simulink model "pacemaker_final"  (R2025a)
settings: Solver=FixedStepAuto  StartTime=0.0  StopTime=10  FixedStep=1e-3  RelTol=1e-3  EnableMultiTasking=on
undefined symbols (not defined in the file): A0, A1, D0, D1, D10, D11, D12, D13, D2, D3, D4, D5, D6, D7, D8, D9, PTA0, PTA1, PTA2, PTB2, PTB23, PTB3, PTB9, PTC16, PTC17, PTC2, PTC3, PTC4, PTD0, PTD1, PTD2, PTD3
libraries: frdmk64flib x20, etargetslib x17, dspstat3 x1
settings Model: ExtModeTrigDuration=5  Creator=School Account  LastModifiedBy=user
settings SolverCC: AlgebraicLoopSolver=TrustRegion
settings OptimizationCC: DefaultParameterBehavior=Inlined  EnhancedBackFolding=on  PassReuseOutputArgsAs=Individual arguments  ZeroExternalMemoryAtStartup=off  ZeroInternalMemoryAtStartup=off  MaxStackSize=64  OptimizeBlockOrder=speed  DifferentSizesBufferReuse=on  OptimizationCustomize=off  EfficientTunableParamExpr=on
settings DebuggingCC: ParameterTunabilityLossMsg=error
settings HardwareCC: ProdBitPerPointer=32.0  ProdBitPerSizeT=32.0  ProdBitPerPtrDiffT=32.0  ProdLargestAtomicInteger=Long  ProdLargestAtomicFloat=Double  ProdWordSize=32.0  ProdHWDeviceType=ARM Compatible->ARM Cortex
settings SFSimCC: MATLABDynamicMemAlloc=off
settings RTWCC: SystemTargetFile=ert.tlc  HardwareBoard=NXP FRDM-K64F  TLCOptions="-aInlineSetEventsForThisBaseRateFcn=TLC_FALSE -aSuppressMultiTaskScheduler=TLC_FALSE  -aRateBasedStepFcn=0"  TemplateMakefile=ert_default_tmf  Toolchain=GNU Tools for ARM Embedded Processors  GPUComputeCapability=3.5  Description=Embedded Coder
settings CodeAppCC: ForceParamTrailComments=on  IgnoreCustomStorageClasses=off  OperatorAnnotations=on  SimulinkDataObjDesc=on  SFDataObjDesc=on  InsertBlockDesc=on
settings ERTTargetCC: ExtModeTransport=4.0  ExtModeStaticAlloc=off  ExtModeMexFile=sendToCommService  ExtModeIntrfLevel=Level1  DynamicArrayContainerType=coder::array

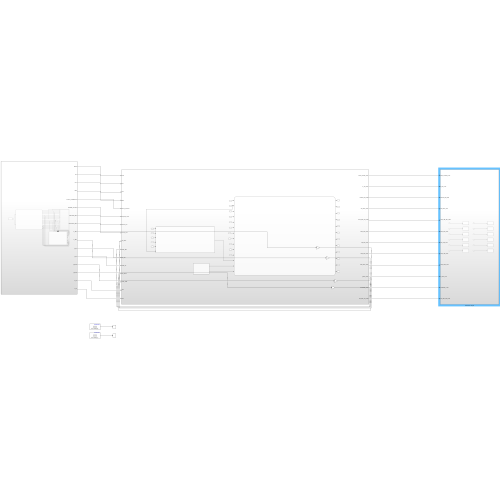
[thumbnail: Simulink's stored preview of the top-level diagram]
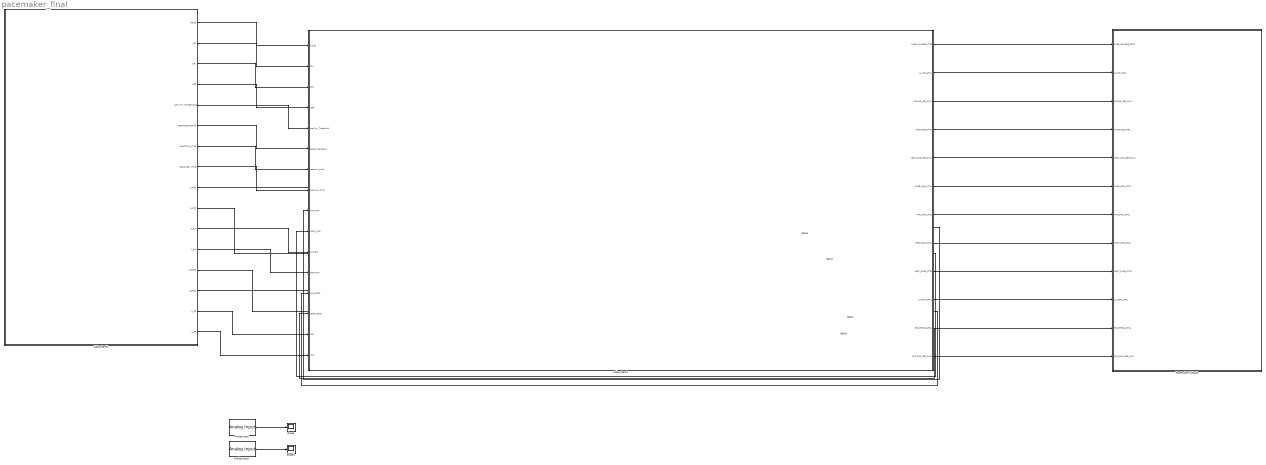
== system pacemaker_final ==
  Analog Input : frdmk64flib/Analog Input  Whichpin=PTB2 (A0)  SampleTime=-1
  Analog Input1 : frdmk64flib/Analog Input  Whichpin=PTB3 (A1)  SampleTime=-1
  Gain1 : Gain  Gain=20
  Gain2 : Gain  Gain=30
  Gain3 : Gain  Gain=30
  Gain4 : Gain  Gain=20
  Pacemaker Outputs : Subsystem
  Scope : Scope
  Scope1 : Scope
      settings: DataLoggingVariableName=ScopeData2
  Subsystem3 : Subsystem
  Subsystem5 : Subsystem
  wires:
  Subsystem3/9(VENT_PACE_CTRL) -> Pacemaker Outputs/9(VENT_PACE_CTRL)
  Subsystem3/8(VENT_GND_CTRL) -> Pacemaker Outputs/8(VENT_GND_CTRL)
  Subsystem3/5(VENT_CMP_REF_PWM) -> Pacemaker Outputs/5(VENT_CMP_REF_PWM)
  Subsystem3/6(PACE_GND_CTRL) -> Pacemaker Outputs/6(PACE_GND_CTRL)
  Subsystem3/3(PACING_REF_PWM) -> Pacemaker Outputs/3(PACING_REF_PWM)
  Subsystem3/4(ATR_PACE_CTRL) -> Pacemaker Outputs/4(ATR_PACE_CTRL)
  Subsystem3/7(ATR_GND_CTRL) -> Pacemaker Outputs/7(ATR_GND_CTRL)
  Subsystem3/10(Z_VENT_CTRL) -> Pacemaker Outputs/10(Z_VENT_CTRL)
  Subsystem3/11(FRONTEND_CTRL) -> Pacemaker Outputs/11(FRONTEND_CTRL)
  Subsystem3/12(ATR_CMP_REF_PWM) -> Pacemaker Outputs/12(ATR_CMP_REF_PWM)
  Subsystem3/1(PACE_CHARGE_CTRL) -> Pacemaker Outputs/1(PACE_CHARGE_CTRL)
  Subsystem3/2(Z_ATR_CTRL) -> Pacemaker Outputs/2(Z_ATR_CTRL)
  Subsystem5/13(A_SENS) -> Gain2/1
  Gain2/1 -> Subsystem3/13(ATR_SENS)
  Subsystem5/9(A_AMP) -> Gain4/1
  Subsystem5/14(V_SENS) -> Gain3/1
  Gain3/1 -> Subsystem3/14(VENT_SENS)
  Subsystem5/11(A_PW) -> Subsystem3/11(ATR_PW)
  Subsystem5/3(URL) -> Subsystem3/3(URL)
  Subsystem5/6(RESPNSE_FACTOR) -> Subsystem3/6(Response_Factor)
  Subsystem5/5(ACTIVITY_THRESHOLD) -> Subsystem3/5(Activity_Threshold)
  Subsystem5/16(V_RP) -> Subsystem3/16(VRP)
  Subsystem5/2(LRL) -> Subsystem3/2(LRL)
  Subsystem5/4(MSR) -> Subsystem3/4(MSR)
  Subsystem5/1(MODE) -> Subsystem3/1(mode)
  Subsystem5/8(RECOVERY_TIME) -> Subsystem3/8(recovery_time)
  Subsystem5/7(REACTION_TIME) -> Subsystem3/7(reaction_time)
  Subsystem5/10(V_AMP) -> Gain1/1
  Gain4/1 -> Subsystem3/9(ATR_AMP)
  Gain1/1 -> Subsystem3/10(VENT_AMP)
  Subsystem5/12(V_PW) -> Subsystem3/12(VENT_PW)
  Subsystem5/15(A_RP) -> Subsystem3/15(ARP)
  Analog Input/1 -> Scope/1
  Analog Input1/1 -> Scope1/1

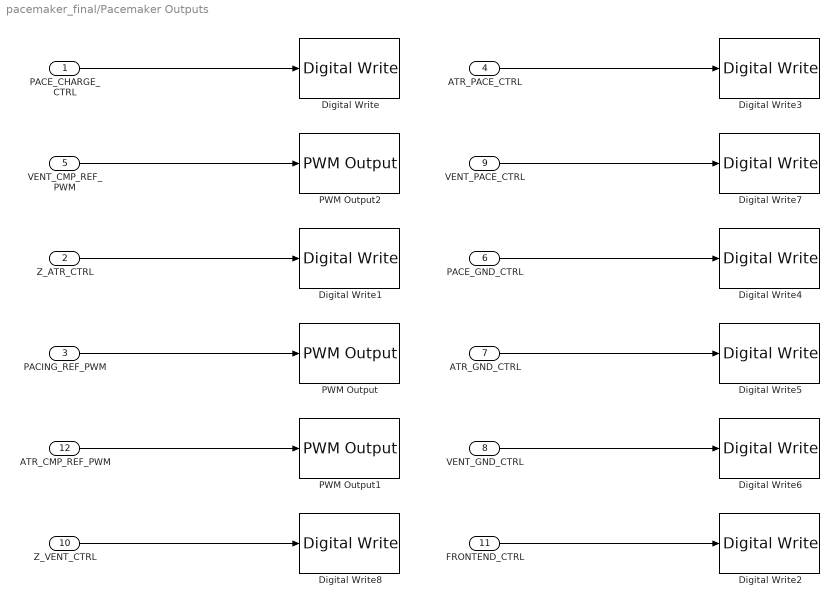
== system pacemaker_final/Pacemaker Outputs ==
  PACE_CHARGE_CTRL : Inport
  Z_ATR_CTRL : Inport  Port=2
  PACING_REF_PWM : Inport  Port=3
  ATR_PACE_CTRL : Inport  Port=4
  VENT_CMP_REF_PWM : Inport  Port=5
  PACE_GND_CTRL : Inport  Port=6
  ATR_GND_CTRL : Inport  Port=7
  VENT_GND_CTRL : Inport  Port=8
  VENT_PACE_CTRL : Inport  Port=9
  Z_VENT_CTRL : Inport  Port=10
  FRONTEND_CTRL : Inport  Port=11
  ATR_CMP_REF_PWM : Inport  Port=12
  Digital Write : frdmk64flib/Digital Write  Whichpin=PTB9 (D2)
  Digital Write1 : frdmk64flib/Digital Write  Whichpin=PTB23 (D4)
  Digital Write2 : frdmk64flib/Digital Write  Whichpin=PTD1 (D13)
  Digital Write3 : frdmk64flib/Digital Write  Whichpin=PTA0 (D8)
  Digital Write4 : frdmk64flib/Digital Write  Whichpin=PTD0 (D10)
  Digital Write5 : frdmk64flib/Digital Write  Whichpin=PTD2 (D11)
  Digital Write6 : frdmk64flib/Digital Write  Whichpin=PTD3 (D12)
  Digital Write7 : frdmk64flib/Digital Write  Whichpin=PTC4 (D9)
  Digital Write8 : frdmk64flib/Digital Write  Whichpin=PTC3 (D7)
  PWM Output : frdmk64flib/PWM Output  Whichpin=PTA2 (D5)  InitialFrequency=2000  InitialDutyCycle=0
  PWM Output1 : frdmk64flib/PWM Output  Whichpin=PTC2 (D6)  InitialFrequency=2000  InitialDutyCycle=0
  PWM Output2 : frdmk64flib/PWM Output  Whichpin=PTA1 (D3)  InitialFrequency=2000  InitialDutyCycle=0
  wires:
  PACE_CHARGE_CTRL/1 -> Digital Write/1
  Z_ATR_CTRL/1 -> Digital Write1/1
  PACING_REF_PWM/1 -> PWM Output/1
  ATR_PACE_CTRL/1 -> Digital Write3/1
  PACE_GND_CTRL/1 -> Digital Write4/1
  ATR_GND_CTRL/1 -> Digital Write5/1
  VENT_GND_CTRL/1 -> Digital Write6/1
  VENT_PACE_CTRL/1 -> Digital Write7/1
  Z_VENT_CTRL/1 -> Digital Write8/1
  FRONTEND_CTRL/1 -> Digital Write2/1
  ATR_CMP_REF_PWM/1 -> PWM Output1/1
  VENT_CMP_REF_PWM/1 -> PWM Output2/1

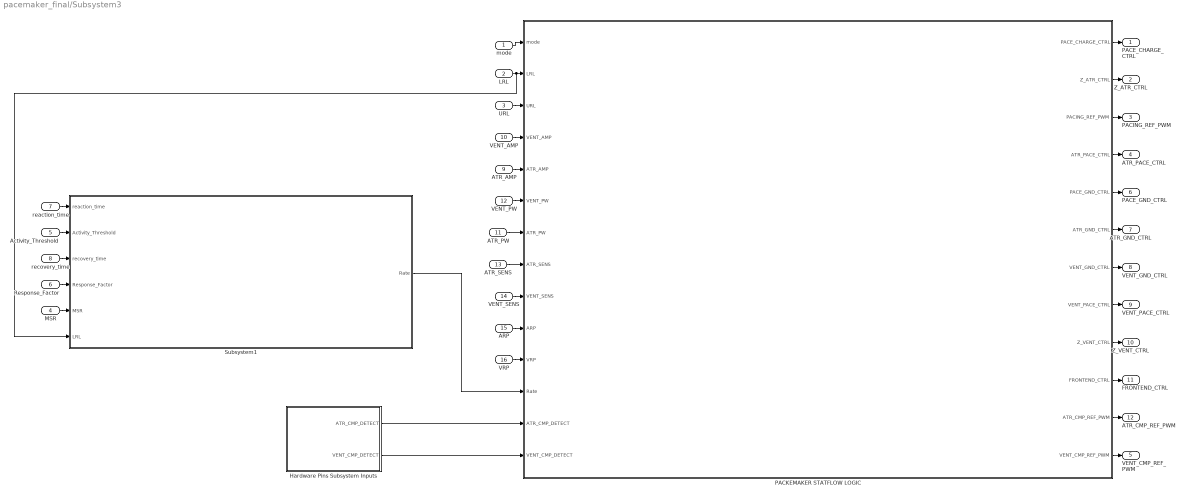
== system pacemaker_final/Subsystem3 ==
  mode : Inport
  LRL : Inport  Port=2
  URL : Inport  Port=3
  MSR : Inport  Port=4
  Activity_Threshold : Inport  Port=5
  Response_Factor : Inport  Port=6
  reaction_time : Inport  Port=7
  recovery_time : Inport  Port=8
  ATR_AMP : Inport  Port=9
  VENT_AMP : Inport  Port=10
  ATR_PW : Inport  Port=11
  VENT_PW : Inport  Port=12
  ATR_SENS : Inport  Port=13
  VENT_SENS : Inport  Port=14
  ARP : Inport  Port=15
  VRP : Inport  Port=16
  Hardware Pins Subsystem Inputs : Subsystem
  PACKEMAKER STATFLOW LOGIC : Stateflow chart  TreatAsAtomicUnit=on
      settings: PortSchema="{\"entries\":[{\"content\":{\"sides\":[{\"content\":{\"connectorIds\":[\"In1\",\"In4\",\"In13\",\"In5\",\"In2\",\"In6\",\"In3\",\"In7\",\"In10\",\"In8\",\"In11\",\"In14\",\"In9\",\"In12\"]},\"type\":\"ConnectorPlacement.EquallySpacedRectSide\",\"uuid\":\"2821f65a-9b3e-4ca7-babd-b0602bfdca31\"},{\"content\":{\"connectorIds\":[\"Out1\",\"Out2\",\"Out3\",\"Out4\",\"Out5\",\"Out6\",\"Out7\",\"Out8\",\"Out9\",\"Out10\",\"Out11\",\"Out12\"],\"side\":\"RIGHT\"},\"type\":\"ConnectorPlacement.EquallySpacedRectSide\",\"uuid\":\"3302ad84-7e85-4bae-9388-240b69681e7f\"},{\"content\":{\"side\":\"TOP\"},\"type\":\"ConnectorPlacement.EquallySpacedRectSide\",\"uuid\":\"cc666da6-1c79-42dc-9f95-9791247ae8bf\"}]},\"type\":\"ConnectorPlacement.EquallySpacedConnector\",\"uuid\":\"e2a43bfa-d126-4f35-adbf-2cf33da0501f\"}],\"packageUris\":[\"http://schema.mathworks.com/mf0/Connector/R2020b\"],\"version\":\"1.0\"}"
  Subsystem1 : Subsystem
  PACE_CHARGE_CTRL : Outport
  Z_ATR_CTRL : Outport  Port=2
  PACING_REF_PWM : Outport  Port=3
  ATR_PACE_CTRL : Outport  Port=4
  VENT_CMP_REF_PWM : Outport  Port=5
  PACE_GND_CTRL : Outport  Port=6
  ATR_GND_CTRL : Outport  Port=7
  VENT_GND_CTRL : Outport  Port=8
  VENT_PACE_CTRL : Outport  Port=9
  Z_VENT_CTRL : Outport  Port=10
  FRONTEND_CTRL : Outport  Port=11
  ATR_CMP_REF_PWM : Outport  Port=12
  wires:
  VENT_PW/1 -> PACKEMAKER STATFLOW LOGIC/6(VENT_PW)
  PACKEMAKER STATFLOW LOGIC/9(Z_VENT_CTRL) -> Z_VENT_CTRL/1
  recovery_time/1 -> Subsystem1/3(recovery_time)
  LRL/1 -> Subsystem1/6(LRL), PACKEMAKER STATFLOW LOGIC/4(LRL)
  PACKEMAKER STATFLOW LOGIC/7(VENT_GND_CTRL) -> VENT_GND_CTRL/1
  Hardware Pins Subsystem Inputs/1(ATR_CMP_DETECT) -> PACKEMAKER STATFLOW LOGIC/9(ATR_CMP_DETECT)
  Response_Factor/1 -> Subsystem1/4(Response_Factor)
  Hardware Pins Subsystem Inputs/2(VENT_CMP_DETECT) -> PACKEMAKER STATFLOW LOGIC/12(VENT_CMP_DETECT)
  Subsystem1/1(Rate) -> PACKEMAKER STATFLOW LOGIC/14(Rate)
  MSR/1 -> Subsystem1/5(MSR)
  PACKEMAKER STATFLOW LOGIC/1(PACE_CHARGE_CTRL) -> PACE_CHARGE_CTRL/1
  Activity_Threshold/1 -> Subsystem1/2(Activity_Threshold)
  PACKEMAKER STATFLOW LOGIC/12(VENT_CMP_REF_PWM) -> VENT_CMP_REF_PWM/1
  PACKEMAKER STATFLOW LOGIC/11(ATR_CMP_REF_PWM) -> ATR_CMP_REF_PWM/1
  reaction_time/1 -> Subsystem1/1(reaction_time)
  PACKEMAKER STATFLOW LOGIC/6(ATR_GND_CTRL) -> ATR_GND_CTRL/1
  PACKEMAKER STATFLOW LOGIC/4(ATR_PACE_CTRL) -> ATR_PACE_CTRL/1
  PACKEMAKER STATFLOW LOGIC/5(PACE_GND_CTRL) -> PACE_GND_CTRL/1
  PACKEMAKER STATFLOW LOGIC/10(FRONTEND_CTRL) -> FRONTEND_CTRL/1
  PACKEMAKER STATFLOW LOGIC/8(VENT_PACE_CTRL) -> VENT_PACE_CTRL/1
  PACKEMAKER STATFLOW LOGIC/3(PACING_REF_PWM) -> PACING_REF_PWM/1
  ATR_SENS/1 -> PACKEMAKER STATFLOW LOGIC/7(ATR_SENS)
  VENT_AMP/1 -> PACKEMAKER STATFLOW LOGIC/5(VENT_AMP)
  ARP/1 -> PACKEMAKER STATFLOW LOGIC/8(ARP)
  VENT_SENS/1 -> PACKEMAKER STATFLOW LOGIC/10(VENT_SENS)
  VRP/1 -> PACKEMAKER STATFLOW LOGIC/11(VRP)
  URL/1 -> PACKEMAKER STATFLOW LOGIC/13(URL)
  PACKEMAKER STATFLOW LOGIC/2(Z_ATR_CTRL) -> Z_ATR_CTRL/1
  mode/1 -> PACKEMAKER STATFLOW LOGIC/1(mode)
  ATR_AMP/1 -> PACKEMAKER STATFLOW LOGIC/2(ATR_AMP)
  ATR_PW/1 -> PACKEMAKER STATFLOW LOGIC/3(ATR_PW)

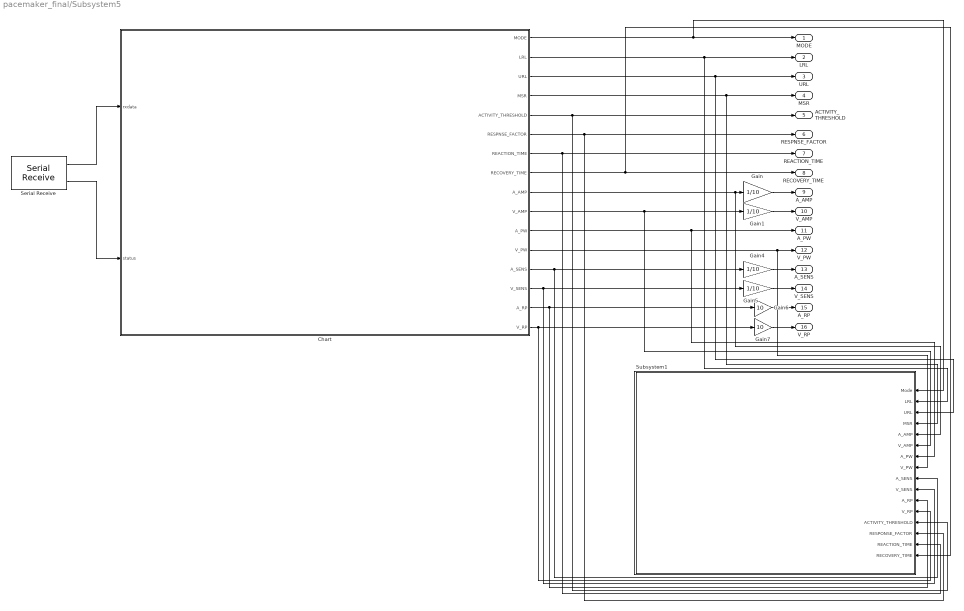
== system pacemaker_final/Subsystem5 ==
  Chart : Stateflow chart  TreatAsAtomicUnit=on
      settings: PortSchema="{\"entries\":[{\"content\":{\"sides\":[{\"content\":{\"connectorIds\":[\"In1\",\"In2\"]},\"type\":\"ConnectorPlacement.EquallySpacedRectSide\",\"uuid\":\"7451ee94-9b00-43e8-b3be-cdc332c766dc\"},{\"content\":{\"connectorIds\":[\"Out6\",\"Out5\",\"Out12\",\"Out7\",\"Out9\",\"Out11\",\"Out8\",\"Out10\",\"Out1\",\"Out13\",\"Out2\",\"Out14\",\"Out4\",\"Out16\",\"Out3\",\"Out15\"],\"side\":\"RIGHT\"},\"type\":\"ConnectorPlacement.EquallySpacedRectSide\",\"uuid\":\"f2d3f72a-cf0a-47d0-b806-afde7d262d5f\"},{\"content\":{\"side\":\"TOP\"},\"type\":\"ConnectorPlacement.EquallySpacedRectSide\",\"uuid\":\"0a90c947-4341-46b5-8896-9140e37675a1\"}]},\"type\":\"ConnectorPlacement.EquallySpacedConnector\",\"uuid\":\"30257972-17b0-4b0b-bedd-1116085aa9d3\"}],\"packageUris\":[\"http://schema.mathworks.com/mf0/Connector/R2020b\"],\"version\":\"1.0\"}"
  Gain{,1,4..5} (4 alike) : Gain  Gain=1/10
  Gain6 : Gain  Gain=10
  Gain7 : Gain  Gain=10
  Serial Receive : frdmk64flib/Serial Receive  SCIModule=0  Baudrate=uint32(9600)  Parity=None  StopBits=1  HardwareFlowControl=None  ByteOrder=LittleEndian  DataType=uint8  DataLength=18  BlockingMode=off  OutputStatus=on  SampleTime=-1
  Subsystem1 : Subsystem
  MODE : Outport
  LRL : Outport  Port=2
  URL : Outport  Port=3
  MSR : Outport  Port=4
  ACTIVITY_THRESHOLD : Outport  Port=5
  RESPNSE_FACTOR : Outport  Port=6
  REACTION_TIME : Outport  Port=7
  RECOVERY_TIME : Outport  Port=8
  A_AMP : Outport  Port=9
  V_AMP : Outport  Port=10
  A_PW : Outport  Port=11
  V_PW : Outport  Port=12
  A_SENS : Outport  Port=13
  V_SENS : Outport  Port=14
  A_RP : Outport  Port=15
  V_RP : Outport  Port=16
  wires:
  Chart/16(V_SENS) -> Subsystem1/10(V_SENS), Gain5/1
  Chart/13(V_AMP) -> Subsystem1/6(V_AMP), Gain1/1
  Chart/1(A_AMP) -> Subsystem1/5(A_AMP), Gain/1
  Serial Receive/1 -> Chart/1(rxdata)
  Chart/3(A_RP) -> Subsystem1/11(A_RP), Gain6/1
  Gain7/1 -> V_RP/1
  Chart/4(A_SENS) -> Subsystem1/9(A_SENS), Gain4/1
  Gain5/1 -> V_SENS/1
  Chart/10(RECOVERY_TIME) -> Subsystem1/16(RECOVERY_TIME), RECOVERY_TIME/1
  Chart/15(V_RP) -> Subsystem1/12(V_RP), Gain7/1
  Chart/2(A_PW) -> A_PW/1, Subsystem1/7(A_PW)
  Chart/11(RESPNSE_FACTOR) -> Subsystem1/14(RESPONSE_FACTOR), RESPNSE_FACTOR/1
  Chart/6(MODE) -> Subsystem1/1(Mode), MODE/1
  Chart/5(LRL) -> Subsystem1/2(LRL), LRL/1
  Chart/9(ACTIVITY_THRESHOLD) -> Subsystem1/13(ACTIVITY_THRESHOLD), ACTIVITY_THRESHOLD/1
  Gain1/1 -> V_AMP/1
  Gain6/1 -> A_RP/1
  Chart/7(MSR) -> Subsystem1/4(MSR), MSR/1
  Chart/14(V_PW) -> V_PW/1, Subsystem1/8(V_PW)
  Chart/12(URL) -> Subsystem1/3(URL), URL/1
  Gain4/1 -> A_SENS/1
  Gain/1 -> A_AMP/1
  Chart/8(REACTION_TIME) -> Subsystem1/15(REACTION_TIME), REACTION_TIME/1
  Serial Receive/2 -> Chart/2(status)

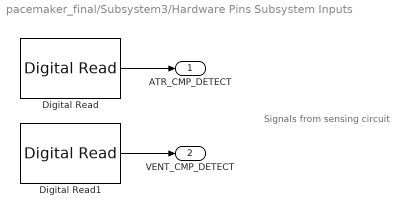
== system pacemaker_final/Subsystem3/Hardware Pins Subsystem Inputs ==
  note: Signals from sensing circuit
  Digital Read : frdmk64flib/Digital Read  Whichpin=PTC16 (D0)  SampleTime=-1
  Digital Read1 : frdmk64flib/Digital Read  Whichpin=PTC17 (D1)  SampleTime=-1
  ATR_CMP_DETECT : Outport
  VENT_CMP_DETECT : Outport  Port=2
  wires:
  Digital Read1/1 -> VENT_CMP_DETECT/1
  Digital Read/1 -> ATR_CMP_DETECT/1

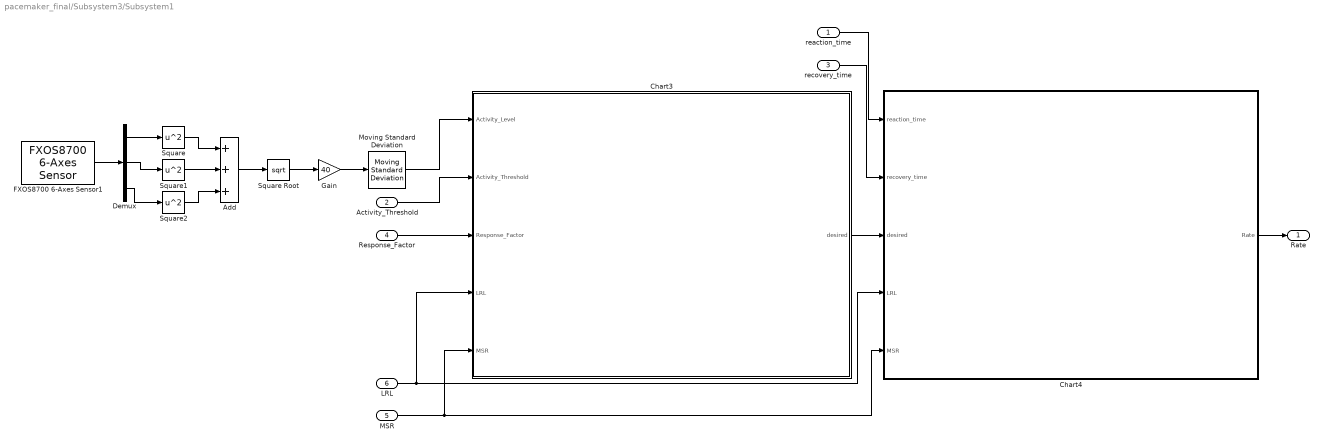
== system pacemaker_final/Subsystem3/Subsystem1 ==
  reaction_time : Inport
  Activity_Threshold : Inport  Port=2
  recovery_time : Inport  Port=3
  Response_Factor : Inport  Port=4
  MSR : Inport  Port=5
  LRL : Inport  Port=6
  Add : Sum  Inputs=+++
  Chart3 : Stateflow chart  TreatAsAtomicUnit=on
  Chart4 : Stateflow chart  TreatAsAtomicUnit=on
      settings: PortSchema="{\"entries\":[{\"content\":{\"sides\":[{\"content\":{\"connectorIds\":[\"In2\",\"In3\",\"In1\",\"In4\",\"In5\"]},\"type\":\"ConnectorPlacement.EquallySpacedRectSide\",\"uuid\":\"edd6887c-315a-49b4-96c6-4b9a398dbb27\"},{\"content\":{\"connectorIds\":[\"Out1\"],\"side\":\"RIGHT\"},\"type\":\"ConnectorPlacement.EquallySpacedRectSide\",\"uuid\":\"e866e153-969a-414b-b9d6-9523e8ffb3f5\"},{\"content\":{\"side\":\"TOP\"},\"type\":\"ConnectorPlacement.EquallySpacedRectSide\",\"uuid\":\"a76f5b9a-cc35-4ca0-a576-c8c761db09b7\"}]},\"type\":\"ConnectorPlacement.EquallySpacedConnector\",\"uuid\":\"7226b5a5-c660-4be3-8454-fc3b1c597f0f\"}],\"packageUris\":[\"http://schema.mathworks.com/mf0/Connector/R2020b\"],\"version\":\"1.0\"}"
  Demux : Demux  Outputs=3
  FXOS8700 6-Axes Sensor1 : frdmk64flib/FXOS8700 6-Axes Sensor  Activesensor=Accelerometer only  ODR=800Hz  HybridODR=400Hz  Accelfullrange=-4g to +4g  SampleTime=0.01
  Gain : Gain  Gain=40
  Moving Standard Deviation : dspstat3/Moving Standard Deviation  Method=Sliding window  ForgettingFactorPort=off  SpecifyWindowLength=on  WindowLength=128  OverlapLength=127  AllowArbitraryInputLength=off  ForgettingFactor=0.9  SimulateUsing=Interpreted execution
  Square : Math  Operator=square
  Square Root : Sqrt
  Square1 : Math  Operator=square
  Square2 : Math  Operator=square
  Rate : Outport
  wires:
  FXOS8700 6-Axes Sensor1/1 -> Demux/1
  Add/1 -> Square Root/1
  Demux/1 -> Square/1
  Demux/2 -> Square1/1
  MSR/1 -> Chart4/5(MSR), Chart3/5(MSR)
  Demux/3 -> Square2/1
  Chart3/1(desired) -> Chart4/1(desired)
  Square/1 -> Add/1
  Square1/1 -> Add/2
  Square2/1 -> Add/3
  Square Root/1 -> Gain/1
  Gain/1 -> Moving Standard Deviation/1
  recovery_time/1 -> Chart4/3(recovery_time)
  Moving Standard Deviation/1 -> Chart3/1(Activity_Level)
  reaction_time/1 -> Chart4/2(reaction_time)
  Activity_Threshold/1 -> Chart3/2(Activity_Threshold)
  Response_Factor/1 -> Chart3/3(Response_Factor)
  LRL/1 -> Chart4/4(LRL), Chart3/4(LRL)
  Chart4/1(Rate) -> Rate/1

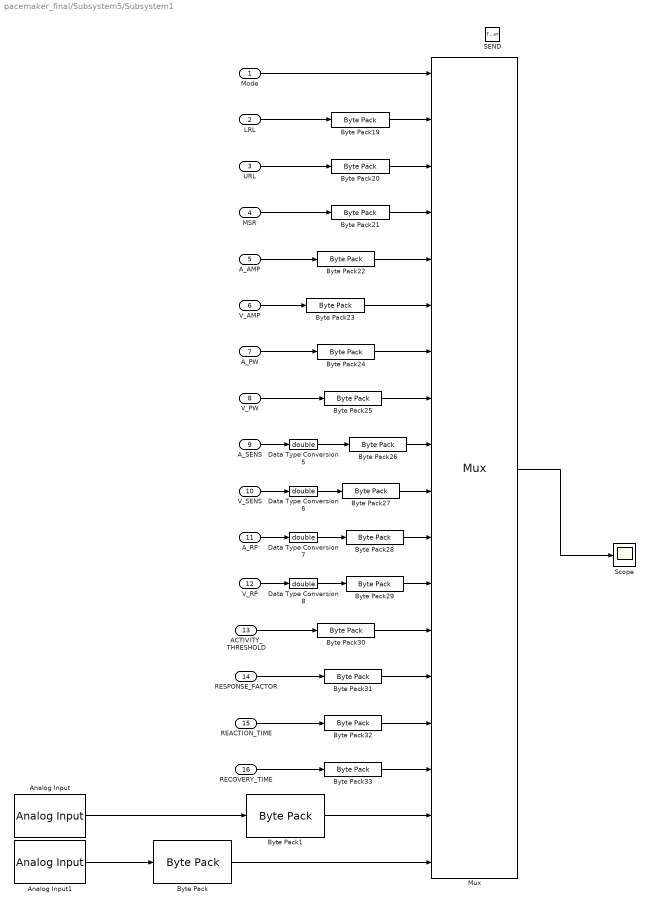
== system pacemaker_final/Subsystem5/Subsystem1 ==
  Mode : Inport
  LRL : Inport  Port=2
  URL : Inport  Port=3
  MSR : Inport  Port=4
  A_AMP : Inport  Port=5
  V_AMP : Inport  Port=6
  A_PW : Inport  Port=7
  V_PW : Inport  Port=8
  A_SENS : Inport  Port=9
  V_SENS : Inport  Port=10
  A_RP : Inport  Port=11
  V_RP : Inport  Port=12
  ACTIVITY_THRESHOLD : Inport  Port=13
  RESPONSE_FACTOR : Inport  Port=14
  REACTION_TIME : Inport  Port=15
  RECOVERY_TIME : Inport  Port=16
  SEND : TriggerPort  TriggerType=function-call  IsSimulinkFunction=on  FunctionName=SEND_PARAM  VariantControl=(inherit)
  Analog Input : frdmk64flib/Analog Input  Whichpin=PTB3 (A1)  SampleTime=-1
  Analog Input1 : frdmk64flib/Analog Input  Whichpin=PTB2 (A0)  SampleTime=-1
  Byte Pack{,1,19..33} (17 alike) : etargetslib/Byte Pack  datatypes={'double'}  byteAlign=1
  Data Type Conversion{5..8} (4 alike) : DataTypeConversion  OutDataTypeStr=double  SaturateOnIntegerOverflow=off  RndMeth=Floor
  Mux : Mux  Inputs=18
  Scope : Scope
  wires:
  Mode/1 -> Mux/1
  Mux/1 -> Scope/1
  LRL/1 -> Byte Pack19/1
  URL/1 -> Byte Pack20/1
  A_AMP/1 -> Byte Pack22/1
  V_AMP/1 -> Byte Pack23/1
  MSR/1 -> Byte Pack21/1
  A_RP/1 -> Data Type Conversion7/1
  V_PW/1 -> Byte Pack25/1
  V_SENS/1 -> Data Type Conversion6/1
  A_SENS/1 -> Data Type Conversion5/1
  A_PW/1 -> Byte Pack24/1
  V_RP/1 -> Data Type Conversion8/1
  RESPONSE_FACTOR/1 -> Byte Pack31/1
  RECOVERY_TIME/1 -> Byte Pack33/1
  REACTION_TIME/1 -> Byte Pack32/1
  ACTIVITY_THRESHOLD/1 -> Byte Pack30/1
  Byte Pack1/1 -> Mux/17
  Analog Input1/1 -> Byte Pack/1
  Byte Pack/1 -> Mux/18
  Analog Input/1 -> Byte Pack1/1
  Byte Pack19/1 -> Mux/2
  Byte Pack20/1 -> Mux/3
  Byte Pack21/1 -> Mux/4
  Byte Pack22/1 -> Mux/5
  Byte Pack23/1 -> Mux/6
  Byte Pack24/1 -> Mux/7
  Byte Pack25/1 -> Mux/8
  Byte Pack26/1 -> Mux/9
  Data Type Conversion5/1 -> Byte Pack26/1
  Data Type Conversion6/1 -> Byte Pack27/1
  Data Type Conversion7/1 -> Byte Pack28/1
  Data Type Conversion8/1 -> Byte Pack29/1
  Byte Pack27/1 -> Mux/10
  Byte Pack28/1 -> Mux/11
  Byte Pack29/1 -> Mux/12
  Byte Pack30/1 -> Mux/13
  Byte Pack31/1 -> Mux/14
  Byte Pack32/1 -> Mux/15
  Byte Pack33/1 -> Mux/16

== stateflow chart pacemaker_final/Subsystem3/PACKEMAKER STATFLOW LOGIC ==
  state Start
  state AOO
    state AOO_Charge
      entry:
      %Charging C22
      ATR_PACE_CTRL = 0;
      VENT_PACE_CTRL = 0;
      PACING_REF_PWM = ATR_AMP;
      PACE_CHARGE_CTRL = 1;
      %Discharging C21
      PACE_GND_CTRL = 1;
      ATR_PACE_CTRL = 0;
      Z_VENT_CTRL = 0;
      Z_ATR_CTRL = 0;
      VENT_PACE_CTRL = 0;
      VENT_GND_CTRL = 0;
      ATR_GND_CTRL = 1;
    state AOO_Pace
      entry:
      %Pacing
      PACE_CHARGE_CTRL = 0;
      PACE_GND_CTRL= 1;
      VENT_PACE_CTRL = 0;
      VENT_GND_CTRL= 0;
      Z_VENT_CTRL = 0;
      Z_ATR_CTRL = 0;
      ATR_GND_CTRL = 0;
      ATR_PACE_CTRL = 1;
    (default) -> AOO.AOO_Charge
    AOO.AOO_Charge -> AOO.AOO_Pace : [after(60000/LRL - ATR_PW,msec)]
    AOO.AOO_Pace -> AOO.AOO_Charge : [after(ATR_PW,msec)]
  state VOO
    state VOO_Charge
      entry:
      %Charging C22
      VENT_PACE_CTRL = 0;
      ATR_PACE_CTRL = 0;
      PACING_REF_PWM = VENT_AMP;
      PACE_CHARGE_CTRL = 1;
      %Discharging C21
      PACE_GND_CTRL = 1;
      VENT_PACE_CTRL = 0;
      Z_ATR_CTRL = 0;
      Z_VENT_CTRL = 0;
      ATR_PACE_CTRL = 0;
      ATR_GND_CTRL = 0;
      VENT_GND_CTRL = 1;
    state AOO_Pace
      entry:
      %Pacing
      PACE_CHARGE_CTRL = 0;
      PACE_GND_CTRL= 1;
      ATR_PACE_CTRL = 0;
      ATR_GND_CTRL= 0;
      Z_ATR_CTRL = 0;
      Z_VENT_CTRL = 0;
      VENT_GND_CTRL = 0;
      VENT_PACE_CTRL = 1;
    (default) -> VOO.VOO_Charge
    VOO.VOO_Charge -> VOO.AOO_Pace : [after(60000/LRL  - VENT_PW,msec)]
    VOO.AOO_Pace -> VOO.VOO_Charge : [after(VENT_PW,msec)]
  state AAI
    state AAI_Charge
      entry:
      FRONTEND_CTRL = 1;
      %Charging C22
      ATR_PACE_CTRL = 0;
      VENT_PACE_CTRL = 0;
      PACING_REF_PWM = ATR_AMP;
      PACE_CHARGE_CTRL = 1;
      %Discharging C21
      PACE_GND_CTRL = 1;
      ATR_PACE_CTRL = 0;
      Z_VENT_CTRL = 0;
      Z_ATR_CTRL = 0;
      VENT_PACE_CTRL = 0;
      VENT_GND_CTRL = 0;
      ATR_GND_CTRL = 1;
      ATR_CMP_REF_PWM = ATR_SENS;
    state AAI_Pace
      entry:
      FRONTEND_CTRL = 0;
      %Pacing
      PACE_CHARGE_CTRL = 0;
      PACE_GND_CTRL= 1;
      VENT_PACE_CTRL = 0;
      VENT_GND_CTRL= 0;
      Z_VENT_CTRL = 0;
      Z_ATR_CTRL = 0;
      ATR_GND_CTRL = 0;
      ATR_PACE_CTRL= 1;
    (default) -> AAI.AAI_Charge
    AAI.AAI_Charge -> AAI.AAI_Pace [order 1] : [after(60000/LRL  - ATR_PW - ARP,msec)]
    AAI.AAI_Pace -> AAI.AAI_Charge : [after( ATR_PW,msec)]
    AAI.AAI_Charge -> (junction 58) [order 2] : [ATR_CMP_DETECT == 1]
    (junction 58) -> (junction 84) : [after(ATR_PW,msec)]
    (junction 84) -> AAI.AAI_Charge : [after(ARP, msec)]
  state VVI
    state VVI_Charge
      entry:
      FRONTEND_CTRL = 1;
      %Charging C22
      VENT_PACE_CTRL = 0;
      ATR_PACE_CTRL = 0;
      PACING_REF_PWM = VENT_AMP;
      PACE_CHARGE_CTRL = 1;
      %Discharging C21
      PACE_GND_CTRL = 1;
      VENT_PACE_CTRL = 0;
      Z_ATR_CTRL = 0;
      Z_VENT_CTRL = 0;
      ATR_PACE_CTRL = 0;
      ATR_GND_CTRL = 0;
      VENT_GND_CTRL = 1;
      VENT_CMP_REF_PWM = VENT_SENS;
    state VVI_Pace
      entry:
      FRONTEND_CTRL = 0;
      %Pacing
      PACE_CHARGE_CTRL = 0;
      PACE_GND_CTRL= 1;
      ATR_PACE_CTRL = 0;
      ATR_GND_CTRL= 0;
      Z_ATR_CTRL = 0;
      Z_VENT_CTRL = 0;
      VENT_GND_CTRL = 0;
      VENT_PACE_CTRL = 1;
    (default) -> VVI.VVI_Charge
    VVI.VVI_Charge -> VVI.VVI_Pace [order 1] : [after(60000/LRL  - VENT_PW - VRP,msec)]
    VVI.VVI_Pace -> VVI.VVI_Charge : [after(VENT_PW,msec)]
    VVI.VVI_Charge -> (junction 65) [order 2] : [VENT_CMP_DETECT == 1]
    (junction 65) -> (junction 82) : [after(VENT_PW,msec)]
    (junction 82) -> VVI.VVI_Charge : [after(VRP, msec)]
  state AOOR
    state AOO_Charge
      entry:
      %Charging C22
      ATR_PACE_CTRL = 0;
      VENT_PACE_CTRL = 0;
      PACING_REF_PWM = ATR_AMP;
      PACE_CHARGE_CTRL = 1;
      %Discharging C21
      PACE_GND_CTRL = 1;
      ATR_PACE_CTRL = 0;
      Z_VENT_CTRL = 0;
      Z_ATR_CTRL = 0;
      VENT_PACE_CTRL = 0;
      VENT_GND_CTRL = 0;
      ATR_GND_CTRL = 1;
    state AOO_Pace
      entry:
      %Pacing
      PACE_CHARGE_CTRL = 0;
      PACE_GND_CTRL= 1;
      VENT_PACE_CTRL = 0;
      VENT_GND_CTRL= 0;
      Z_VENT_CTRL = 0;
      Z_ATR_CTRL = 0;
      ATR_GND_CTRL = 0;
      ATR_PACE_CTRL = 1;
    (default) -> AOOR.AOO_Charge
    AOOR.AOO_Charge -> AOOR.AOO_Pace : [after(60000/Rate - ATR_PW,msec)]
    AOOR.AOO_Pace -> AOOR.AOO_Charge : [after(ATR_PW,msec)]
  state VOOR
    state VOO_Charge
      entry:
      %Charging C22
      VENT_PACE_CTRL = 0;
      ATR_PACE_CTRL = 0;
      PACING_REF_PWM = VENT_AMP;
      PACE_CHARGE_CTRL = 1;
      %Discharging C21
      PACE_GND_CTRL = 1;
      VENT_PACE_CTRL = 0;
      Z_ATR_CTRL = 0;
      Z_VENT_CTRL = 0;
      ATR_PACE_CTRL = 0;
      ATR_GND_CTRL = 0;
      VENT_GND_CTRL = 1;
    state AOO_Pace
      entry:
      %Pacing
      PACE_CHARGE_CTRL = 0;
      PACE_GND_CTRL= 1;
      ATR_PACE_CTRL = 0;
      ATR_GND_CTRL= 0;
      Z_ATR_CTRL = 0;
      Z_VENT_CTRL = 0;
      VENT_GND_CTRL = 0;
      VENT_PACE_CTRL = 1;
    (default) -> VOOR.VOO_Charge
    VOOR.VOO_Charge -> VOOR.AOO_Pace : [after(60000/Rate - VENT_PW,msec)]
    VOOR.AOO_Pace -> VOOR.VOO_Charge : [after(VENT_PW,msec)]
  state AAIR
    state AAI_Charge
      entry:
      FRONTEND_CTRL = 1;
      %Charging C22
      ATR_PACE_CTRL = 0;
      VENT_PACE_CTRL = 0;
      PACING_REF_PWM = ATR_AMP;
      PACE_CHARGE_CTRL = 1;
      %Discharging C21
      PACE_GND_CTRL = 1;
      ATR_PACE_CTRL = 0;
      Z_VENT_CTRL = 0;
      Z_ATR_CTRL = 0;
      VENT_PACE_CTRL = 0;
      VENT_GND_CTRL = 0;
      ATR_GND_CTRL = 1;
      ATR_CMP_REF_PWM = ATR_SENS;
    state AAI_Pace
      entry:
      FRONTEND_CTRL = 0;
      %Pacing
      PACE_CHARGE_CTRL = 0;
      PACE_GND_CTRL= 1;
      VENT_PACE_CTRL = 0;
      VENT_GND_CTRL= 0;
      Z_VENT_CTRL = 0;
      Z_ATR_CTRL = 0;
      ATR_GND_CTRL = 0;
      ATR_PACE_CTRL= 1;
    (default) -> AAIR.AAI_Charge
    AAIR.AAI_Charge -> AAIR.AAI_Pace [order 1] : [after(60000/Rate - ATR_PW - ARP,msec)]
    AAIR.AAI_Pace -> AAIR.AAI_Charge : [after( ATR_PW,msec)]
    AAIR.AAI_Charge -> (junction 107) [order 2] : [ATR_CMP_DETECT == 1]
    (junction 107) -> (junction 108) : [after(ATR_PW,msec)]
    (junction 108) -> AAIR.AAI_Charge : [after(ARP, msec)]
  state VVIR
    state VVI_Charge
      entry:
      FRONTEND_CTRL = 1;
      %Charging C22
      VENT_PACE_CTRL = 0;
      ATR_PACE_CTRL = 0;
      PACING_REF_PWM = VENT_AMP;
      PACE_CHARGE_CTRL = 1;
      %Discharging C21
      PACE_GND_CTRL = 1;
      VENT_PACE_CTRL = 0;
      Z_ATR_CTRL = 0;
      Z_VENT_CTRL = 0;
      ATR_PACE_CTRL = 0;
      ATR_GND_CTRL = 0;
      VENT_GND_CTRL = 1;
      VENT_CMP_REF_PWM = VENT_SENS;
    state VVI_Pace
      entry:
      FRONTEND_CTRL = 0;
      %Pacing
      PACE_CHARGE_CTRL = 0;
      PACE_GND_CTRL= 1;
      ATR_PACE_CTRL = 0;
      ATR_GND_CTRL= 0;
      Z_ATR_CTRL = 0;
      Z_VENT_CTRL = 0;
      VENT_GND_CTRL = 0;
      VENT_PACE_CTRL = 1;
    (default) -> VVIR.VVI_Charge
    VVIR.VVI_Charge -> VVIR.VVI_Pace [order 1] : [after(60000/Rate - VENT_PW - VRP,msec)]
    VVIR.VVI_Pace -> VVIR.VVI_Charge : [after(VENT_PW,msec)]
    VVIR.VVI_Charge -> (junction 118) [order 2] : [VENT_CMP_DETECT == 1]
    (junction 118) -> (junction 119) : [after(VENT_PW,msec)]
    (junction 119) -> VVIR.VVI_Charge : [after(VRP, msec)]
  (default) -> Start
  AOO -> Start : [mode ~= 1]
  Start -> AOO [order 2] : [mode == 1]
  Start -> VOO [order 1] : [mode == 2]
  VOO -> Start : [mode ~= 2]
  Start -> AAI [order 3] : [mode == 3]
  AAI -> Start : [mode ~= 3]
  Start -> VVI [order 4] : [mode == 4]
  VVI -> Start : [mode ~= 4]
  Start -> AOOR [order 5] : [mode == 5]
  AOOR -> Start : [mode ~= 5]
  Start -> VOOR [order 6] : [mode == 6]
  VOOR -> Start : [mode ~= 6]
  Start -> AAIR [order 7] : [mode == 7]
  AAIR -> Start : [mode ~= 7]
  Start -> VVIR [order 8] : [mode == 8]
  VVIR -> Start : [mode ~= 8]
  data: PACE_CHARGE_CTRL output; Z_ATR_CTRL output; PACING_REF_PWM output; mode input; ATR_PACE_CTRL output; PACE_GND_CTRL output; ATR_AMP input; ATR_GND_CTRL output; ATR_PW input; LRL input; VENT_AMP input; VENT_GND_CTRL output; VENT_PACE_CTRL output; Z_VENT_CTRL output; VENT_PW input; FRONTEND_CTRL output; ATR_CMP_REF_PWM output; ATR_SENS input; ARP input; ATR_CMP_DETECT input; VENT_SENS input; VENT_CMP_REF_PWM output; VRP input; VENT_CMP_DETECT input; URL input; Rate input

== stateflow chart pacemaker_final/Subsystem3/Subsystem1/Chart3 ==
  state intial
    entry:
    desired=LRL
  state Break
  state Function
    during:
    scaled = Response_Factor * (Activity_Level - Activity_Threshold)
    desired = LRL + scaled
    if desired > MSR
    desired = MSR;
    elseif desired < LRL
    desired = LRL;
    end
  (default) -> intial
  intial -> Break
  Function -> Break : [Activity_Level < Activity_Threshold]
  Break -> Function : [Activity_Level >= Activity_Threshold]
  data: Activity_Level input; Activity_Threshold input; Response_Factor input; desired output; scaled local; LRL input; MSR input

== stateflow chart pacemaker_final/Subsystem3/Subsystem1/Chart4 ==
  state Intial
    entry:
    Rate=LRL
  state Rates
    during:
    pace_up   = (MSR - LRL) / reaction_time*1
    pace_down = (MSR - LRL) / recovery_time*1
  state Pace_Up
    during:
    Rate=Rate+pace_up
    if (Rate>MSR)
    Rate=MSR;
    end
  state Pace_Down
    during:
    Rate = Rate - pace_down;
    if (Rate<LRL)
    Rate = LRL;
    end
  (default) -> Intial
  Intial -> Rates
  Rates -> Pace_Up [order 2] : [Rate<desired]
  Rates -> Pace_Down [order 1] : [Rate>desired]
  Pace_Down -> Rates : [Rate<=desired]
  Pace_Up -> Rates : [Rate>=desired]
  data: desired input; reaction_time input; recovery_time input; Rate output; pace_down local; pace_up local; LRL input; MSR input

== stateflow chart pacemaker_final/Subsystem5/Chart ==
  state SET_PARAM
    entry:
    MODE = rxdata(3)
    LRL = double(rxdata(4))
    URL = double(rxdata(5))
    MSR = double(rxdata(6))
    A_AMP = double(rxdata(7))
    V_AMP = double(rxdata(8))
    A_PW = double(rxdata(9))
    V_PW = double(rxdata(10))
    A_SENS = double(rxdata(11))
    V_SENS = double(rxdata(12))
    V_RP = double(rxdata(13))
    A_RP = double(rxdata(14))
    ACTIVITY_THRESHOLD = double(rxdata(15))
    REACTION_TIME = double(rxdata(16))
    RESPNSE_FACTOR = double(rxdata(17))
    RECOVERY_TIME = double(rxdata(18))
  state Intial
    entry:
    MODE = 1 %uint8
    LRL = 60 %uint8
    URL = 120 %uint8
    MSR = 120 %uint8
    A_AMP = 35 %single /10
    V_AMP = 35 %single /10
    A_PW = 4 %single /10 ms
    V_PW = 4 %single /10 ms
    A_SENS = 0 %single /10
    V_SENS = 0 %single /10
    V_RP = 32 %uint16 *100
    A_RP =  25 %uint16 *100
    ACTIVITY_THRESHOLD = 0 %uint8
    REACTION_TIME = 30 %uint8 secs
    RESPNSE_FACTOR = 8 %uint8
    RECOVERY_TIME = 5 %uint8 mins
  state STANDBY
  state ECHO_PARAM
    entry:
    SEND_PARAM();
  SET_PARAM -> STANDBY
  (junction 25) -> SET_PARAM [order 2] : [rxdata(2) == hex2dec('55')]
  (default) -> Intial
  (junction 28) -> STANDBY [order 2]
  Intial -> STANDBY
  (junction 28) -> (junction 25) [order 1] : [rxdata(1) == hex2dec('16')]
  STANDBY -> (junction 28) : [status == 0]
  (junction 25) -> ECHO_PARAM [order 1] : [rxdata(2) == hex2dec('22')]
  ECHO_PARAM -> STANDBY
  data: A_AMP output; A_PW output; A_RP output; A_SENS output; LRL output; MODE output; MSR output; REACTION_TIME output; ACTIVITY_THRESHOLD output; RECOVERY_TIME output; RESPNSE_FACTOR output; URL output; V_AMP output; V_PW output; V_RP output; V_SENS output; rxdata input; status input
